simulink model "Modelling_Sim"  (R2017b)
settings: Solver=VariableStepAuto  StartTime=0.0  StopTime=50  RelTol=1e-3
settings Model: Creator=Oguzhan  LastModifiedBy=Oguzhan

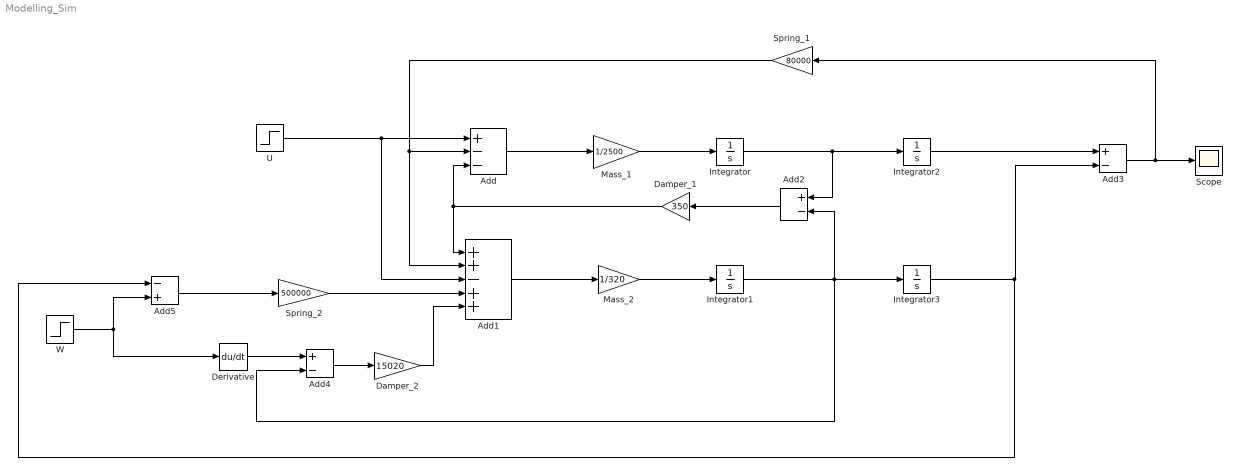
== system Modelling_Sim ==
  Add : Sum  Inputs=+--
  Add1 : Sum  Inputs=++-++
  Add2 : Sum  Inputs=+-
  Add3 : Sum  Inputs=+-
  Add4 : Sum  Inputs=+-
  Add5 : Sum  Inputs=-+
  Damper_1 : Gain  Gain=350
  Damper_2 : Gain  Gain=15020
  Derivative : Derivative
  Integrator{,1..3} (4 alike) : Integrator
  Mass_1 : Gain  Gain=1/2500
  Mass_2 : Gain  Gain=1/320
  Scope : Scope
  Spring_1 : Gain  Gain=80000
  Spring_2 : Gain  Gain=500000
  "U " : Step  Time=0  SampleTime=0
  W : Step  Time=0  After=0.0  SampleTime=0
  wires:
  Add/1 -> Mass_1/1
  Mass_1/1 -> Integrator/1
  Add1/1 -> Mass_2/1
  Mass_2/1 -> Integrator1/1
  Integrator/1 -> Add2/1, Integrator2/1
  Add2/1 -> Damper_1/1
  Integrator1/1 -> Add4/2, Integrator3/1, Add2/2
  Damper_1/1 -> Add/3, Add1/1
  Integrator2/1 -> Add3/1
  Integrator3/1 -> Add5/1, Add3/2
  Add4/1 -> Damper_2/1
  Derivative/1 -> Add4/1
  W/1 -> Derivative/1, Add5/2
  Add5/1 -> Spring_2/1
  Spring_2/1 -> Add1/4
  Damper_2/1 -> Add1/5
  Add3/1 -> Spring_1/1, Scope/1
  Spring_1/1 -> Add/2, Add1/2
  "U "/1 -> Add1/3, Add/1
